simulink model "Plant2"  (R2016b)
settings: Solver=VariableStepAuto  StartTime=0.0  StopTime=200  FixedStep=0.001  RelTol=1e-3  EnableMultiTasking=on
libraries: fuzblock x1
settings Model: Creator=Huu Toan  LastModifiedBy=Truc
settings DataIOCC: LimitDataPoints=on  SaveFormat=Array  SignalLoggingSaveFormat=ModelDataLogs
settings OptimizationCC: InitFltsAndDblsToZero=on  LifeSpan=inf
settings DebuggingCC: SaveWithParameterizedLinksMsg=none  UnderspecifiedInitializationDetection=Classic  MergeDetectMultiDrivingBlocksExec=none  SignalResolutionControl=TryResolveAllWithWarning  SolverPrmCheckMsg=warning  MultiTaskDSMMsg=warning  MultiTaskCondExecSysMsg=none  SFUnexpectedBacktrackingDiag=warning  SFNoUnconditionalDefaultTransitionDiag=warning  SFExecutionAtInitializationDiag=none
settings HardwareCC: ProdBitPerPointer=32  ProdBitPerSizeT=32  ProdBitPerPtrDiffT=32  ProdLargestAtomicFloat=None  ProdIntDivRoundTo=Undefined  ProdEndianess=Unspecified  ProdWordSize=32  ProdHWDeviceType=32-bit Generic
settings ModelReferenceCC: PropagateSignalLabelsOutOfModel=off
settings GRTTargetCC: TargetFcnLib=ansi_tfl_tmw.mat  TargetLangStandard=C89/C90 (ANSI)  CombineOutputUpdateFcns=off  GRTInterface=on
settings ConfigComp: CovMetricSettings=dw  CovHtmlReporting=on  CovSaveCumulativeToWorkspaceVar=on  CovSaveSingleToWorkspaceVar=on  CovExternalEMLEnable=off

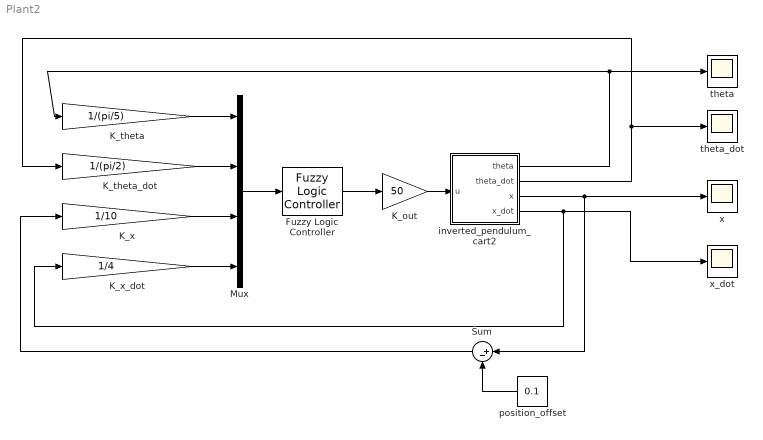
== system Plant2 ==
  Fuzzy Logic Controller : fuzblock/Fuzzy Logic  Controller  fis='invertedPendulumCart.fis'
  K_out : Gain  Gain=50
  K_theta : Gain  Gain=1/(pi/5)
  K_theta_dot : Gain  Gain=1/(pi/2)
  K_x : Gain  Gain=1/10
  K_x_dot : Gain  Gain=1/4
  Mux : Mux
  Sum : Sum  Inputs=|+-
  inverted_pendulum_cart2 : Subsystem  mask{M=2.5, I=0.05, m_=0.01, L=0.7, g=0.98, init_cond=[pi/6 0 0.3 0]}
      mask prompts: M "Cart mass (M)"; I "Moment (I)"; m_ "Pendulum mass (m)"; L "Pendulum length (L)"; g "Gravity (g)"; init_cond "Initial Condition"
  position_offset : Constant  Value=0.1
  theta : Scope
  theta_dot : Scope
  x : Scope
  x_dot : Scope
  wires:
  inverted_pendulum_cart2/1(theta) -> theta/1, K_theta/1
  inverted_pendulum_cart2/2(theta_dot) -> theta_dot/1, K_theta_dot/1
  inverted_pendulum_cart2/3(x) -> x/1, Sum/1
  inverted_pendulum_cart2/4(x_dot) -> x_dot/1, K_x_dot/1
  K_theta/1 -> Mux/1
  K_x/1 -> Mux/3
  K_theta_dot/1 -> Mux/2
  K_out/1 -> inverted_pendulum_cart2/1(u)
  Mux/1 -> Fuzzy Logic Controller/1
  Fuzzy Logic Controller/1 -> K_out/1
  K_x_dot/1 -> Mux/4
  position_offset/1 -> Sum/2
  Sum/1 -> K_x/1

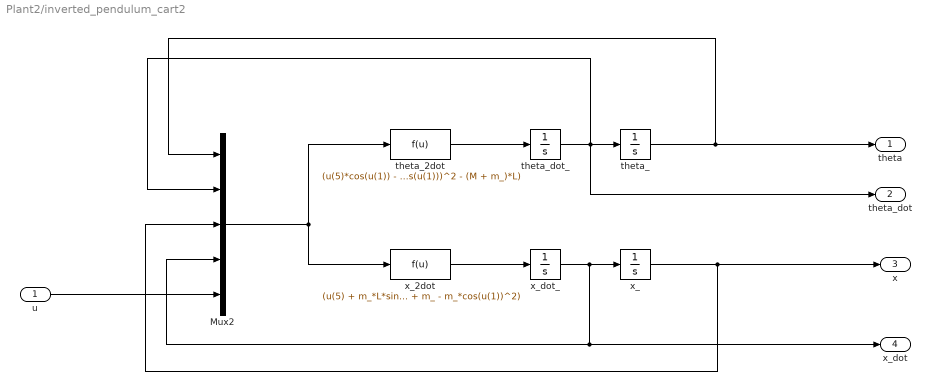
== system Plant2/inverted_pendulum_cart2 ==
  u : Inport
  Mux2 : Mux  Inputs=5
  theta_ : Integrator  InitialCondition=init_cond(1)
  theta_2dot : Fcn  Expr=(u(5)*cos(u(1)) - (M + m_)*g*sin(u(1)) + m_*L*cos(u(1))*sin(u(1))*u(2)) / (m_*L*(cos(u(1)))^2 - (M + m_)*L)
  theta_dot_ : Integrator  InitialCondition=init_cond(2)
  x_ : Integrator  InitialCondition=init_cond(3)
  x_2dot : Fcn  Expr=(u(5) + m_*L*sin(u(1))*u(2)^2 - m_*g*cos(u(1))*sin(u(1))) / (M + m_ - m_*cos(u(1))^2)
  x_dot_ : Integrator  InitialCondition=init_cond(4)
  theta : Outport
  theta_dot : Outport  Port=2
  x : Outport  Port=3
  x_dot : Outport  Port=4
  wires:
  x_/1 -> Mux2/3, x/1
  x_dot_/1 -> Mux2/4, x_dot/1, x_/1
  theta_/1 -> Mux2/1, theta/1
  theta_dot_/1 -> theta_dot/1, Mux2/2, theta_/1
  theta_2dot/1 -> theta_dot_/1
  x_2dot/1 -> x_dot_/1
  Mux2/1 -> x_2dot/1, theta_2dot/1
  u/1 -> Mux2/5
